simulink library "WECSim_Lib"  (R2014b)
settings: Solver=ode45  StartTime=0.0  StopTime=10.0  RelTol=1e-3
undefined symbols (not defined in the file): body, constraint, pto, simu, waves, X, Y, Z
libraries: nesl_utility x178, sm_lib x59, vrlib x12
(part 3 of 6)

== system WECSim_Lib/PTOs/Translational PTO (Local X) ==
  note: pto.loc
      | pto.c
      | pto.k
  note: Constraints the motion to the desired DOF.
      | Applies PTO loads to the body based on PTO restoring and damping values.
      | Moves the connection points (B and F) from the free surface to the PTO location.
      | Calculates the PTO internal mecahnics force and power.
      | Outputs motions, forces, and power.
  Assignment{,1..3} (4 alike) : Assignment  DiagnosticForDimensions=Warning
  "Assignment (1st index) " : Assignment
  Assignment (1st index)1 : Assignment
  Assignment (1st index)2 : Assignment
  Assignment (1st index)3 : Assignment
  Bus Creator1 : BusCreator  Inputs=8
  Constant{,1..3} (4 alike) : Constant  Value=[0 0 0 0 0 0]
  ForceAndPower : Subsystem
  Gai1 : Gain  Gain=-1
  Gai57 : Gain  Gain=-1
  Gain4 : Gain  Gain=-1
  Gain5 : Gain  Gain=-1
  Mux1 : Mux  Inputs=2
  Mux3 : Mux  Inputs=2
  PS-Simulink Converter{,1..7} (8 alike) : nesl_utility/PS-Simulink Converter  PhysicalDomain=network_engine_domain  SubClassName=ps_output  LeftPortType=input  RightPortType=output  PseudoPeriodic=off  Frequencies=[]  Unit=1  AffineConversion=off
  Rigid Transform : sm_lib/Frames and Transforms/Rigid Transform  TranslationMethod=Cartesian  TranslationLengthUnit=m  TranslationStandardAxis=+Z  TranslationStandardOffset=0  TranslationCartesianOffset=pto.loc  TranslationROffset=0  TranslationROffsetUnits=m  TranslationZOffset=0  TranslationZOffsetUnits=m  TranslationThetaOffset=0  TranslationThetaOffsetUnits=deg  RotationMethod=StandardAxis  RotationAngleUnits=deg  RotationStandardAxis=+Y  RotationAngle=90  RotationArbitraryAxis=[0 0 1]  FollAlignAxisA=+X  BaseAlignAxisA=+Y  FollAlignAxisB=+Y  BaseAlignAxisB=+Z  RotationMatrix=[1 0 0; 0 1 0; 0 0 1]  BlockFunction=simmechanics.library.frames_transforms.rigid_transform
  Rigid Transform1 : sm_lib/Frames and Transforms/Rigid Transform  TranslationMethod=Cartesian  TranslationLengthUnit=m  TranslationStandardAxis=+Z  TranslationStandardOffset=0  TranslationCartesianOffset=pto.loc  TranslationROffset=0  TranslationROffsetUnits=m  TranslationZOffset=0  TranslationZOffsetUnits=m  TranslationThetaOffset=0  TranslationThetaOffsetUnits=deg  RotationMethod=StandardAxis  RotationAngleUnits=deg  RotationStandardAxis=+Y  RotationAngle=90  RotationArbitraryAxis=[0 0 1]  FollAlignAxisA=+X  BaseAlignAxisA=+Y  FollAlignAxisB=+Y  BaseAlignAxisB=+Z  RotationMatrix=[1 0 0; 0 1 0; 0 0 1]  BlockFunction=simmechanics.library.frames_transforms.rigid_transform
  Selector{,2,4,6} (4 alike) : Selector  InputPortWidth=3  Indices=[3 2 1]
  Selector{1,3,5,7} (4 alike) : Selector  InputPortWidth=3  Indices=[3]
  Translational PCC (Prismatic Joint) : sm_lib/Joints/Prismatic Joint  SenseConstraintForce=on  SenseConstraintForceX=off  SenseConstraintForceY=off  SenseConstraintForceZ=off  SenseConstraintTorque=on  SenseConstraintTorqueX=off  SenseConstraintTorqueY=off  SenseConstraintTorqueZ=off  SenseTotalForce=on  SenseTotalForceX=off  SenseTotalForceY=off  SenseTotalForceZ=off  SenseTotalTorque=on  SenseTotalTorqueX=off  SenseTotalTorqueY=off  SenseTotalTorqueZ=off  CompositeWrenchDir=BaseOnFollower  CompositeWrenchFrame=BaseFrame  EquilibriumPosition=0  EquilibriumPositionUnits=m  SpringStiffness=pto.k  SpringStiffnessUnits=N/m  DampingCoefficient=pto.c  DampingCoefficientUnits=N/(m/s)  TorqueActuationMode=NoTorque  MotionActuationMode=ComputedMotion  SensePosition=on  SenseVelocity=on  SenseAcceleration=on  SenseTorqueForce=on  PositionTargetValue=0  PositionTargetValueUnits=m  PositionTargetSpecify=off  PositionTargetPriority=High  VelocityTargetValue=0  VelocityTargetValueUnits=m/s  VelocityTargetSpecify=off  VelocityTargetPriority=High  BlockFunction=simmechanics.library.joints.prismatic_joint
  output : ToWorkspace  VariableName=pto1_out  SaveFormat=Structure With Time  SampleTime=-1
      settings: Decimation=round(simu.dtOut/simu.dt,0)
  F : PMIOPort  Port=1  Side=Left
  B : PMIOPort  Port=2  Side=Right
  wires:
  Selector2/1 -> Selector3/1, Assignment/1
  Selector3/1 -> Gai57/1
  Gai57/1 -> Assignment/2
  Selector/1 -> Selector1/1, Assignment1/1
  Selector1/1 -> Gain4/1
  Gain4/1 -> Assignment1/2
  ForceAndPower/2(Power) -> Bus Creator1/8  "powerInternalMechanics"
  ForceAndPower/1(Force) -> Bus Creator1/7  "forceInternalMechanics"
  Assignment (1st index)2/1 -> Bus Creator1/3  "acceleration"
  Assignment (1st index)1/1 -> ForceAndPower/2(Vel), Bus Creator1/2  "velocity"
  "Assignment (1st index) "/1 -> ForceAndPower/1(Pos), Bus Creator1/1  "position"
  Assignment (1st index)3/1 -> Bus Creator1/5  "forceActuation"
  Mux3/1 -> Bus Creator1/4  "forceTotal"
  Mux1/1 -> Bus Creator1/6  "forceConstraint"
  Bus Creator1/1 -> output/1
  PS-Simulink Converter4/1 -> Selector/1
  PS-Simulink Converter5/1 -> Selector2/1
  Constant/1 -> "Assignment (1st index) "/1
  PS-Simulink Converter/1 -> "Assignment (1st index) "/2
  Constant1/1 -> Assignment (1st index)1/1
  PS-Simulink Converter1/1 -> Assignment (1st index)1/2
  Constant2/1 -> Assignment (1st index)2/1
  Constant3/1 -> Assignment (1st index)3/1
  PS-Simulink Converter2/1 -> Assignment (1st index)2/2
  PS-Simulink Converter3/1 -> Assignment (1st index)3/2
  Assignment1/1 -> Mux1/1
  Assignment/1 -> Mux1/2
  Selector6/1 -> Assignment2/1, Selector7/1
  Selector7/1 -> Gai1/1
  Gai1/1 -> Assignment2/2
  Selector4/1 -> Assignment3/1, Selector5/1
  Selector5/1 -> Gain5/1
  Gain5/1 -> Assignment3/2
  PS-Simulink Converter6/1 -> Selector4/1
  PS-Simulink Converter7/1 -> Selector6/1
  Assignment3/1 -> Mux3/1
  Assignment2/1 -> Mux3/2
  connections:
  Rigid Transform/LConn1 -- B/RConn1
  Rigid Transform/RConn1 -- Translational PCC (Prismatic Joint)/LConn1
  Rigid Transform1/LConn1 -- F/RConn1
  PS-Simulink Converter4/LConn1 -- Translational PCC (Prismatic Joint)/RConn6
  PS-Simulink Converter5/LConn1 -- Translational PCC (Prismatic Joint)/RConn7
  Translational PCC (Prismatic Joint)/RConn2 -- PS-Simulink Converter/LConn1
  Translational PCC (Prismatic Joint)/RConn3 -- PS-Simulink Converter1/LConn1
  Translational PCC (Prismatic Joint)/RConn4 -- PS-Simulink Converter2/LConn1
  Translational PCC (Prismatic Joint)/RConn1 -- Rigid Transform1/RConn1
  Translational PCC (Prismatic Joint)/RConn5 -- PS-Simulink Converter3/LConn1
  Translational PCC (Prismatic Joint)/RConn8 -- PS-Simulink Converter6/LConn1
  PS-Simulink Converter7/LConn1 -- Translational PCC (Prismatic Joint)/RConn9

== system WECSim_Lib/PTOs/Translational PTO (Local Z) ==
  note: pto.loc
      | pto.c
      | pto.k
  note: Constraints the motion to the desired DOF.
      | Applies PTO loads to the body based on PTO restoring and damping values.
      | Moves the connection points (B and F) from the free surface to the PTO location.
      | Calculates the PTO internal mecahnics force and power.
      | Outputs motions, forces, and power.
  "Assignment (3rd index) " : Assignment  Indices=3
  Assignment (3rd index)1 : Assignment  Indices=3
  Assignment (3rd index)2 : Assignment  Indices=3
  Assignment (3rd index)3 : Assignment  Indices=3
  Bus Creator1 : BusCreator  Inputs=8
  Constant{,1..3} (4 alike) : Constant  Value=[0 0 0 0 0 0]
  InternalMechanics : Subsystem
  Mux1 : Mux  Inputs=2
  Mux4 : Mux  Inputs=2
  PS-Simulink Converter{,1..7} (8 alike) : nesl_utility/PS-Simulink Converter  PhysicalDomain=network_engine_domain  SubClassName=ps_output  LeftPortType=input  RightPortType=output  PseudoPeriodic=off  Frequencies=[]  Unit=1  AffineConversion=off
  Rigid Transform : sm_lib/Frames and Transforms/Rigid Transform  TranslationMethod=Cartesian  TranslationLengthUnit=m  TranslationStandardAxis=+Z  TranslationStandardOffset=0  TranslationCartesianOffset=pto.loc  TranslationROffset=0  TranslationROffsetUnits=m  TranslationZOffset=0  TranslationZOffsetUnits=m  TranslationThetaOffset=0  TranslationThetaOffsetUnits=deg  RotationMethod=None  RotationAngleUnits=deg  RotationStandardAxis=+X  RotationAngle=90  RotationArbitraryAxis=[0 0 1]  FollAlignAxisA=+X  BaseAlignAxisA=+Y  FollAlignAxisB=+Y  BaseAlignAxisB=+Z  RotationMatrix=[1 0 0; 0 1 0; 0 0 1]  BlockFunction=simmechanics.library.frames_transforms.rigid_transform
  Rigid Transform1 : sm_lib/Frames and Transforms/Rigid Transform  TranslationMethod=Cartesian  TranslationLengthUnit=m  TranslationStandardAxis=+Z  TranslationStandardOffset=0  TranslationCartesianOffset=pto.loc  TranslationROffset=0  TranslationROffsetUnits=m  TranslationZOffset=0  TranslationZOffsetUnits=m  TranslationThetaOffset=0  TranslationThetaOffsetUnits=deg  RotationMethod=None  RotationAngleUnits=deg  RotationStandardAxis=+X  RotationAngle=90  RotationArbitraryAxis=[0 0 1]  FollAlignAxisA=+X  BaseAlignAxisA=+Y  FollAlignAxisB=+Y  BaseAlignAxisB=+Z  RotationMatrix=[1 0 0; 0 1 0; 0 0 1]  BlockFunction=simmechanics.library.frames_transforms.rigid_transform
  Translational PCC (Prismatic Joint) : sm_lib/Joints/Prismatic Joint  SenseConstraintForce=on  SenseConstraintForceX=off  SenseConstraintForceY=off  SenseConstraintForceZ=off  SenseConstraintTorque=on  SenseConstraintTorqueX=off  SenseConstraintTorqueY=off  SenseConstraintTorqueZ=off  SenseTotalForce=on  SenseTotalForceX=off  SenseTotalForceY=off  SenseTotalForceZ=off  SenseTotalTorque=on  SenseTotalTorqueX=off  SenseTotalTorqueY=off  SenseTotalTorqueZ=off  CompositeWrenchDir=BaseOnFollower  CompositeWrenchFrame=BaseFrame  EquilibriumPosition=0  EquilibriumPositionUnits=m  SpringStiffness=pto.k  SpringStiffnessUnits=N/m  DampingCoefficient=pto.c  DampingCoefficientUnits=N/(m/s)  TorqueActuationMode=NoTorque  MotionActuationMode=ComputedMotion  SensePosition=on  SenseVelocity=on  SenseAcceleration=on  SenseTorqueForce=on  PositionTargetValue=0  PositionTargetValueUnits=m  PositionTargetSpecify=off  PositionTargetPriority=High  VelocityTargetValue=0  VelocityTargetValueUnits=m/s  VelocityTargetSpecify=off  VelocityTargetPriority=High  BlockFunction=simmechanics.library.joints.prismatic_joint
  output : ToWorkspace  VariableName=pto1_out  SaveFormat=Structure With Time  SampleTime=-1
      settings: Decimation=round(simu.dtOut/simu.dt,0)
  F : PMIOPort  Port=1  Side=Left
  B : PMIOPort  Port=2  Side=Right
  wires:
  Bus Creator1/1 -> output/1
  Mux1/1 -> Bus Creator1/6  "forceConstraint"
  Mux4/1 -> Bus Creator1/4  "forceTotal"
  PS-Simulink Converter4/1 -> Mux1/1
  PS-Simulink Converter5/1 -> Mux1/2
  PS-Simulink Converter6/1 -> Mux4/1
  PS-Simulink Converter7/1 -> Mux4/2
  Assignment (3rd index)3/1 -> Bus Creator1/5  "forceActuation"
  "Assignment (3rd index) "/1 -> InternalMechanics/1(Position), Bus Creator1/1  "position"
  Assignment (3rd index)1/1 -> InternalMechanics/2(Velocity), Bus Creator1/2  "velocity"
  Assignment (3rd index)2/1 -> Bus Creator1/3  "acceleration"
  Constant/1 -> "Assignment (3rd index) "/1
  PS-Simulink Converter/1 -> "Assignment (3rd index) "/2
  Constant1/1 -> Assignment (3rd index)1/1
  PS-Simulink Converter1/1 -> Assignment (3rd index)1/2
  Constant2/1 -> Assignment (3rd index)2/1
  PS-Simulink Converter2/1 -> Assignment (3rd index)2/2
  InternalMechanics/1(Force) -> Bus Creator1/7  "forceInternalMechanics"
  InternalMechanics/2(Power) -> Bus Creator1/8  "powerInternalMechanics"
  Constant3/1 -> Assignment (3rd index)3/1
  PS-Simulink Converter3/1 -> Assignment (3rd index)3/2  "forceActuation"
  connections:
  Rigid Transform/RConn1 -- Translational PCC (Prismatic Joint)/LConn1
  B/RConn1 -- Rigid Transform/LConn1
  Translational PCC (Prismatic Joint)/RConn5 -- PS-Simulink Converter3/LConn1
  Translational PCC (Prismatic Joint)/RConn9 -- PS-Simulink Converter7/LConn1
  Translational PCC (Prismatic Joint)/RConn1 -- Rigid Transform1/RConn1
  Translational PCC (Prismatic Joint)/RConn4 -- PS-Simulink Converter2/LConn1
  Translational PCC (Prismatic Joint)/RConn7 -- PS-Simulink Converter5/LConn1
  Translational PCC (Prismatic Joint)/RConn3 -- PS-Simulink Converter1/LConn1
  Rigid Transform1/LConn1 -- F/RConn1
  Translational PCC (Prismatic Joint)/RConn8 -- PS-Simulink Converter6/LConn1
  Translational PCC (Prismatic Joint)/RConn2 -- PS-Simulink Converter/LConn1
  Translational PCC (Prismatic Joint)/RConn6 -- PS-Simulink Converter4/LConn1

== system WECSim_Lib/PTOs/Translational PTO Prescribed Motion (Local X) ==
  note: Constraints the motion to the desired DOF.
      | Applies PTO loads to the body based on PTO restoring and damping values.
      | Additionally forces User Defined motions, and outputs required actuation force.
      | Moves the connection points (B and F) from the free surface to the PTO location.
      | Calculates the PTO internal mecahnics force and power.
      | Outputs motions, forces, and power.
  note: pto.loc
      | pto.c
      | pto.k
  position : Inport
  velocity : Inport  Port=2
  acceleration : Inport  Port=3
  Assignment{,1..3} (4 alike) : Assignment  DiagnosticForDimensions=Warning
  "Assignment (1st index) " : Assignment
  Assignment (1st index)1 : Assignment
  Assignment (1st index)2 : Assignment
  Assignment (1st index)3 : Assignment
  Bus Creator1 : BusCreator  Inputs=8
  Constant{,1..3} (4 alike) : Constant  Value=[0 0 0 0 0 0]
  ForceAndPower : Subsystem
  Gai1 : Gain  Gain=-1
  Gai57 : Gain  Gain=-1
  Gain4 : Gain  Gain=-1
  Gain5 : Gain  Gain=-1
  Mux1 : Mux  Inputs=2
  Mux3 : Mux  Inputs=2
  PS-Simulink Converter{,1..7} (8 alike) : nesl_utility/PS-Simulink Converter  PhysicalDomain=network_engine_domain  SubClassName=ps_output  LeftPortType=input  RightPortType=output  PseudoPeriodic=off  Frequencies=[]  Unit=1  AffineConversion=off
  Rigid Transform : sm_lib/Frames and Transforms/Rigid Transform  TranslationMethod=Cartesian  TranslationLengthUnit=m  TranslationStandardAxis=+Z  TranslationStandardOffset=0  TranslationCartesianOffset=pto.loc  TranslationROffset=0  TranslationROffsetUnits=m  TranslationZOffset=0  TranslationZOffsetUnits=m  TranslationThetaOffset=0  TranslationThetaOffsetUnits=deg  RotationMethod=StandardAxis  RotationAngleUnits=deg  RotationStandardAxis=+Y  RotationAngle=90  RotationArbitraryAxis=[0 0 1]  FollAlignAxisA=+X  BaseAlignAxisA=+Y  FollAlignAxisB=+Y  BaseAlignAxisB=+Z  RotationMatrix=[1 0 0; 0 1 0; 0 0 1]  BlockFunction=simmechanics.library.frames_transforms.rigid_transform
  Rigid Transform1 : sm_lib/Frames and Transforms/Rigid Transform  TranslationMethod=Cartesian  TranslationLengthUnit=m  TranslationStandardAxis=+Z  TranslationStandardOffset=0  TranslationCartesianOffset=pto.loc  TranslationROffset=0  TranslationROffsetUnits=m  TranslationZOffset=0  TranslationZOffsetUnits=m  TranslationThetaOffset=0  TranslationThetaOffsetUnits=deg  RotationMethod=StandardAxis  RotationAngleUnits=deg  RotationStandardAxis=+Y  RotationAngle=90  RotationArbitraryAxis=[0 0 1]  FollAlignAxisA=+X  BaseAlignAxisA=+Y  FollAlignAxisB=+Y  BaseAlignAxisB=+Z  RotationMatrix=[1 0 0; 0 1 0; 0 0 1]  BlockFunction=simmechanics.library.frames_transforms.rigid_transform
  Selector{,2,4,6} (4 alike) : Selector  InputPortWidth=3  Indices=[3 2 1]
  Selector{1,3,5,7} (4 alike) : Selector  InputPortWidth=3  Indices=[3]
  Simulink-PS Converter : nesl_utility/Simulink-PS Converter  PhysicalDomain=network_engine_domain  SubClassName=ps_input  LeftPortType=input  RightPortType=output  PseudoPeriodic=off  Frequencies=[]  NoiseDistribution=none  NoiseParameters=[]  Unit=1  AffineConversion=off  InputFiltering=derivs  SimscapeFilterOrder=2  InputFilterTimeConstant=0.001  UdotUserProvided=2
  Translational PCC (Prismatic Joint) : sm_lib/Joints/Prismatic Joint  SenseConstraintForce=on  SenseConstraintForceX=off  SenseConstraintForceY=off  SenseConstraintForceZ=off  SenseConstraintTorque=on  SenseConstraintTorqueX=off  SenseConstraintTorqueY=off  SenseConstraintTorqueZ=off  SenseTotalForce=on  SenseTotalForceX=off  SenseTotalForceY=off  SenseTotalForceZ=off  SenseTotalTorque=on  SenseTotalTorqueX=off  SenseTotalTorqueY=off  SenseTotalTorqueZ=off  CompositeWrenchDir=BaseOnFollower  CompositeWrenchFrame=BaseFrame  EquilibriumPosition=0  EquilibriumPositionUnits=m  SpringStiffness=pto.k  SpringStiffnessUnits=N/m  DampingCoefficient=pto.c  DampingCoefficientUnits=N/(m/s)  TorqueActuationMode=ComputedTorque  MotionActuationMode=InputMotion  SensePosition=on  SenseVelocity=on  SenseAcceleration=on  SenseTorqueForce=on  PositionTargetValue=0  PositionTargetValueUnits=m  PositionTargetSpecify=off  PositionTargetPriority=High  VelocityTargetValue=0  VelocityTargetValueUnits=m/s  VelocityTargetSpecify=off  VelocityTargetPriority=High  BlockFunction=simmechanics.library.joints.prismatic_joint
  output : ToWorkspace  VariableName=pto1_out  SaveFormat=Structure With Time  SampleTime=-1
      settings: Decimation=round(simu.dtOut/simu.dt,0)
  F : PMIOPort  Port=1  Side=Left
  B : PMIOPort  Port=2  Side=Right
  wires:
  acceleration/1 -> Simulink-PS Converter/3
  velocity/1 -> Simulink-PS Converter/2
  position/1 -> Simulink-PS Converter/1
  Assignment2/1 -> Mux3/2
  Assignment3/1 -> Mux3/1
  PS-Simulink Converter7/1 -> Selector6/1
  PS-Simulink Converter6/1 -> Selector4/1
  Gain5/1 -> Assignment3/2
  Selector5/1 -> Gain5/1
  Selector4/1 -> Selector5/1, Assignment3/1
  Gai1/1 -> Assignment2/2
  Selector7/1 -> Gai1/1
  Selector6/1 -> Selector7/1, Assignment2/1
  Assignment/1 -> Mux1/2
  Assignment1/1 -> Mux1/1
  PS-Simulink Converter3/1 -> Assignment (1st index)3/2
  PS-Simulink Converter2/1 -> Assignment (1st index)2/2
  Constant3/1 -> Assignment (1st index)3/1
  Constant2/1 -> Assignment (1st index)2/1
  PS-Simulink Converter1/1 -> Assignment (1st index)1/2
  Constant1/1 -> Assignment (1st index)1/1
  PS-Simulink Converter/1 -> "Assignment (1st index) "/2
  Constant/1 -> "Assignment (1st index) "/1
  PS-Simulink Converter5/1 -> Selector2/1
  PS-Simulink Converter4/1 -> Selector/1
  Bus Creator1/1 -> output/1
  Mux1/1 -> Bus Creator1/6  "forceConstraint"
  Mux3/1 -> Bus Creator1/4  "forceTotal"
  Assignment (1st index)3/1 -> Bus Creator1/5  "forceActuation"
  ForceAndPower/1(Force) -> Bus Creator1/7  "forceInternalMechanics"
  ForceAndPower/2(Power) -> Bus Creator1/8  "powerInternalMechanics"
  Gain4/1 -> Assignment1/2
  Selector1/1 -> Gain4/1
  Selector/1 -> Assignment1/1, Selector1/1
  Gai57/1 -> Assignment/2
  Selector3/1 -> Gai57/1
  Selector2/1 -> Assignment/1, Selector3/1
  "Assignment (1st index) "/1 -> ForceAndPower/1(Pos), Bus Creator1/1  "position"
  Assignment (1st index)1/1 -> ForceAndPower/2(Vel), Bus Creator1/2  "velocity"
  Assignment (1st index)2/1 -> Bus Creator1/3  "acceleration"
  connections:
  Simulink-PS Converter/RConn1 -- Translational PCC (Prismatic Joint)/LConn2
  PS-Simulink Converter7/LConn1 -- Translational PCC (Prismatic Joint)/RConn9
  Translational PCC (Prismatic Joint)/RConn8 -- PS-Simulink Converter6/LConn1
  Translational PCC (Prismatic Joint)/RConn5 -- PS-Simulink Converter3/LConn1
  Translational PCC (Prismatic Joint)/RConn1 -- Rigid Transform1/RConn1
  Translational PCC (Prismatic Joint)/RConn4 -- PS-Simulink Converter2/LConn1
  Translational PCC (Prismatic Joint)/RConn3 -- PS-Simulink Converter1/LConn1
  Translational PCC (Prismatic Joint)/RConn2 -- PS-Simulink Converter/LConn1
  PS-Simulink Converter5/LConn1 -- Translational PCC (Prismatic Joint)/RConn7
  PS-Simulink Converter4/LConn1 -- Translational PCC (Prismatic Joint)/RConn6
  Rigid Transform1/LConn1 -- F/RConn1
  Rigid Transform/RConn1 -- Translational PCC (Prismatic Joint)/LConn1
  Rigid Transform/LConn1 -- B/RConn1

== system WECSim_Lib/PTOs/Translational PTO Prescribed Motion (Local Z) ==
  note: Constraints the motion to the desired DOF.
      | Applies PTO loads to the body based on PTO restoring and damping values.
      | Additionally forces User Defined motions, and outputs required actuation force.
      | Moves the connection points (B and F) from the free surface to the PTO location.
      | Calculates the PTO internal mecahnics force and power.
      | Outputs motions, forces, and power.
  note: pto.loc
      | pto.c
      | pto.k
  position : Inport
  velocity : Inport  Port=2
  acceleration : Inport  Port=3
  "Assignment (3rd index) " : Assignment  Indices=3
  Assignment (3rd index)1 : Assignment  Indices=3
  Assignment (3rd index)2 : Assignment  Indices=3
  Assignment (3rd index)3 : Assignment  Indices=3
  Bus Creator1 : BusCreator  Inputs=8
  Constant{,1..3} (4 alike) : Constant  Value=[0 0 0 0 0 0]
  InternalMechanics : Subsystem
  Mux1 : Mux  Inputs=2
  Mux4 : Mux  Inputs=2
  PS-Simulink Converter{,1..7} (8 alike) : nesl_utility/PS-Simulink Converter  PhysicalDomain=network_engine_domain  SubClassName=ps_output  LeftPortType=input  RightPortType=output  PseudoPeriodic=off  Frequencies=[]  Unit=1  AffineConversion=off
  Rigid Transform : sm_lib/Frames and Transforms/Rigid Transform  TranslationMethod=Cartesian  TranslationLengthUnit=m  TranslationStandardAxis=+Z  TranslationStandardOffset=0  TranslationCartesianOffset=pto.loc  TranslationROffset=0  TranslationROffsetUnits=m  TranslationZOffset=0  TranslationZOffsetUnits=m  TranslationThetaOffset=0  TranslationThetaOffsetUnits=deg  RotationMethod=None  RotationAngleUnits=deg  RotationStandardAxis=+X  RotationAngle=90  RotationArbitraryAxis=[0 0 1]  FollAlignAxisA=+X  BaseAlignAxisA=+Y  FollAlignAxisB=+Y  BaseAlignAxisB=+Z  RotationMatrix=[1 0 0; 0 1 0; 0 0 1]  BlockFunction=simmechanics.library.frames_transforms.rigid_transform
  Rigid Transform1 : sm_lib/Frames and Transforms/Rigid Transform  TranslationMethod=Cartesian  TranslationLengthUnit=m  TranslationStandardAxis=+Z  TranslationStandardOffset=0  TranslationCartesianOffset=pto.loc  TranslationROffset=0  TranslationROffsetUnits=m  TranslationZOffset=0  TranslationZOffsetUnits=m  TranslationThetaOffset=0  TranslationThetaOffsetUnits=deg  RotationMethod=None  RotationAngleUnits=deg  RotationStandardAxis=+X  RotationAngle=90  RotationArbitraryAxis=[0 0 1]  FollAlignAxisA=+X  BaseAlignAxisA=+Y  FollAlignAxisB=+Y  BaseAlignAxisB=+Z  RotationMatrix=[1 0 0; 0 1 0; 0 0 1]  BlockFunction=simmechanics.library.frames_transforms.rigid_transform
  Simulink-PS Converter : nesl_utility/Simulink-PS Converter  PhysicalDomain=network_engine_domain  SubClassName=ps_input  LeftPortType=input  RightPortType=output  PseudoPeriodic=off  Frequencies=[]  NoiseDistribution=none  NoiseParameters=[]  Unit=1  AffineConversion=off  InputFiltering=derivs  SimscapeFilterOrder=2  InputFilterTimeConstant=0.001  UdotUserProvided=2
  Translational PCC (Prismatic Joint) : sm_lib/Joints/Prismatic Joint  SenseConstraintForce=on  SenseConstraintForceX=off  SenseConstraintForceY=off  SenseConstraintForceZ=off  SenseConstraintTorque=on  SenseConstraintTorqueX=off  SenseConstraintTorqueY=off  SenseConstraintTorqueZ=off  SenseTotalForce=on  SenseTotalForceX=off  SenseTotalForceY=off  SenseTotalForceZ=off  SenseTotalTorque=on  SenseTotalTorqueX=off  SenseTotalTorqueY=off  SenseTotalTorqueZ=off  CompositeWrenchDir=BaseOnFollower  CompositeWrenchFrame=BaseFrame  EquilibriumPosition=0  EquilibriumPositionUnits=m  SpringStiffness=pto.k  SpringStiffnessUnits=N/m  DampingCoefficient=pto.c  DampingCoefficientUnits=N/(m/s)  TorqueActuationMode=ComputedTorque  MotionActuationMode=InputMotion  SensePosition=on  SenseVelocity=on  SenseAcceleration=on  SenseTorqueForce=on  PositionTargetValue=0  PositionTargetValueUnits=m  PositionTargetSpecify=off  PositionTargetPriority=High  VelocityTargetValue=0  VelocityTargetValueUnits=m/s  VelocityTargetSpecify=off  VelocityTargetPriority=High  BlockFunction=simmechanics.library.joints.prismatic_joint
  output : ToWorkspace  VariableName=pto1_out  SaveFormat=Structure With Time  SampleTime=-1
      settings: Decimation=round(simu.dtOut/simu.dt,0)
  F : PMIOPort  Port=1  Side=Left
  B : PMIOPort  Port=2  Side=Right
  wires:
  acceleration/1 -> Simulink-PS Converter/3
  velocity/1 -> Simulink-PS Converter/2
  position/1 -> Simulink-PS Converter/1
  Bus Creator1/1 -> output/1
  Mux1/1 -> Bus Creator1/6  "forceConstraint"
  Mux4/1 -> Bus Creator1/4  "forceTotal"
  PS-Simulink Converter4/1 -> Mux1/1
  PS-Simulink Converter5/1 -> Mux1/2
  PS-Simulink Converter6/1 -> Mux4/1
  PS-Simulink Converter7/1 -> Mux4/2
  Assignment (3rd index)3/1 -> Bus Creator1/5  "forceActuation"
  "Assignment (3rd index) "/1 -> InternalMechanics/1(Position), Bus Creator1/1  "position"
  Assignment (3rd index)1/1 -> InternalMechanics/2(Velocity), Bus Creator1/2  "velocity"
  Assignment (3rd index)2/1 -> Bus Creator1/3  "acceleration"
  Constant/1 -> "Assignment (3rd index) "/1
  PS-Simulink Converter/1 -> "Assignment (3rd index) "/2
  Constant1/1 -> Assignment (3rd index)1/1
  PS-Simulink Converter1/1 -> Assignment (3rd index)1/2
  Constant2/1 -> Assignment (3rd index)2/1
  PS-Simulink Converter2/1 -> Assignment (3rd index)2/2
  InternalMechanics/1(Force) -> Bus Creator1/7  "forceInternalMechanics"
  InternalMechanics/2(Power) -> Bus Creator1/8  "powerInternalMechanics"
  Constant3/1 -> Assignment (3rd index)3/1
  PS-Simulink Converter3/1 -> Assignment (3rd index)3/2  "forceActuation"
  connections:
  Translational PCC (Prismatic Joint)/LConn2 -- Simulink-PS Converter/RConn1
  Rigid Transform1/LConn1 -- F/RConn1
  Translational PCC (Prismatic Joint)/RConn1 -- Rigid Transform1/RConn1
  Rigid Transform/RConn1 -- Translational PCC (Prismatic Joint)/LConn1
  B/RConn1 -- Rigid Transform/LConn1
  Translational PCC (Prismatic Joint)/RConn2 -- PS-Simulink Converter/LConn1
  Translational PCC (Prismatic Joint)/RConn3 -- PS-Simulink Converter1/LConn1
  Translational PCC (Prismatic Joint)/RConn4 -- PS-Simulink Converter2/LConn1
  Translational PCC (Prismatic Joint)/RConn5 -- PS-Simulink Converter3/LConn1
  Translational PCC (Prismatic Joint)/RConn6 -- PS-Simulink Converter4/LConn1
  Translational PCC (Prismatic Joint)/RConn7 -- PS-Simulink Converter5/LConn1
  Translational PCC (Prismatic Joint)/RConn8 -- PS-Simulink Converter6/LConn1
  Translational PCC (Prismatic Joint)/RConn9 -- PS-Simulink Converter7/LConn1

== system WECSim_Lib/PTOs/Translational PTO UD Force (Local X) ==
  note: Constraints the motion to the desired DOF.
      | Applies PTO loads to the body based on PTO restoring and damping values.
      | Additionally applies user defined PTO force and outputs PTO position,velocity and acceleration.
      | Moves the connection points (B and F) from the free surface to the PTO location.
      | Calculates the PTO internal mecahnics force and power.
      | Outputs motions, forces, and power.
  note: pto.loc
      | pto.c
      | pto.k
  Torque : Inport
  Assignment{,1..3} (4 alike) : Assignment  DiagnosticForDimensions=Warning
  "Assignment (1st index) " : Assignment
  Assignment (1st index)1 : Assignment
  Assignment (1st index)2 : Assignment
  Assignment (1st index)3 : Assignment
  Bus Creator1 : BusCreator  Inputs=8
  Bus Creator2 : BusCreator  Inputs=3
  Constant{,1..3} (4 alike) : Constant  Value=[0 0 0 0 0 0]
  ForceAndPower : Subsystem
  Gai1 : Gain  Gain=-1
  Gai57 : Gain  Gain=-1
  Gain4 : Gain  Gain=-1
  Gain5 : Gain  Gain=-1
  Mux1 : Mux  Inputs=2
  Mux3 : Mux  Inputs=2
  PS-Simulink Converter{,1..7} (8 alike) : nesl_utility/PS-Simulink Converter  PhysicalDomain=network_engine_domain  SubClassName=ps_output  LeftPortType=input  RightPortType=output  PseudoPeriodic=off  Frequencies=[]  Unit=1  AffineConversion=off
  Rigid Transform : sm_lib/Frames and Transforms/Rigid Transform  TranslationMethod=Cartesian  TranslationLengthUnit=m  TranslationStandardAxis=+Z  TranslationStandardOffset=0  TranslationCartesianOffset=pto.loc  TranslationROffset=0  TranslationROffsetUnits=m  TranslationZOffset=0  TranslationZOffsetUnits=m  TranslationThetaOffset=0  TranslationThetaOffsetUnits=deg  RotationMethod=StandardAxis  RotationAngleUnits=deg  RotationStandardAxis=+Y  RotationAngle=90  RotationArbitraryAxis=[0 0 1]  FollAlignAxisA=+X  BaseAlignAxisA=+Y  FollAlignAxisB=+Y  BaseAlignAxisB=+Z  RotationMatrix=[1 0 0; 0 1 0; 0 0 1]  BlockFunction=simmechanics.library.frames_transforms.rigid_transform
  Rigid Transform1 : sm_lib/Frames and Transforms/Rigid Transform  TranslationMethod=Cartesian  TranslationLengthUnit=m  TranslationStandardAxis=+Z  TranslationStandardOffset=0  TranslationCartesianOffset=pto.loc  TranslationROffset=0  TranslationROffsetUnits=m  TranslationZOffset=0  TranslationZOffsetUnits=m  TranslationThetaOffset=0  TranslationThetaOffsetUnits=deg  RotationMethod=StandardAxis  RotationAngleUnits=deg  RotationStandardAxis=+Y  RotationAngle=90  RotationArbitraryAxis=[0 0 1]  FollAlignAxisA=+X  BaseAlignAxisA=+Y  FollAlignAxisB=+Y  BaseAlignAxisB=+Z  RotationMatrix=[1 0 0; 0 1 0; 0 0 1]  BlockFunction=simmechanics.library.frames_transforms.rigid_transform
  Selector{,2,4,6} (4 alike) : Selector  InputPortWidth=3  Indices=[3 2 1]
  Selector{1,3,5,7} (4 alike) : Selector  InputPortWidth=3  Indices=[3]
  Simulink-PS Converter : nesl_utility/Simulink-PS Converter  PhysicalDomain=network_engine_domain  SubClassName=ps_input  LeftPortType=input  RightPortType=output  PseudoPeriodic=off  Frequencies=[]  NoiseDistribution=none  NoiseParameters=[]  Unit=1  AffineConversion=off  InputFiltering=off  SimscapeFilterOrder=1  InputFilterTimeConstant=0.001  UdotUserProvided=1
  Translational PCC (Prismatic Joint) : sm_lib/Joints/Prismatic Joint  SenseConstraintForce=on  SenseConstraintForceX=off  SenseConstraintForceY=off  SenseConstraintForceZ=off  SenseConstraintTorque=on  SenseConstraintTorqueX=off  SenseConstraintTorqueY=off  SenseConstraintTorqueZ=off  SenseTotalForce=on  SenseTotalForceX=off  SenseTotalForceY=off  SenseTotalForceZ=off  SenseTotalTorque=on  SenseTotalTorqueX=off  SenseTotalTorqueY=off  SenseTotalTorqueZ=off  CompositeWrenchDir=BaseOnFollower  CompositeWrenchFrame=BaseFrame  EquilibriumPosition=0  EquilibriumPositionUnits=m  SpringStiffness=pto.k  SpringStiffnessUnits=N/m  DampingCoefficient=pto.c  DampingCoefficientUnits=N/(m/s)  TorqueActuationMode=InputTorque  MotionActuationMode=ComputedMotion  SensePosition=on  SenseVelocity=on  SenseAcceleration=on  SenseTorqueForce=on  PositionTargetValue=0  PositionTargetValueUnits=m  PositionTargetSpecify=off  PositionTargetPriority=High  VelocityTargetValue=0  VelocityTargetValueUnits=m/s  VelocityTargetSpecify=off  VelocityTargetPriority=High  BlockFunction=simmechanics.library.joints.prismatic_joint
  output : ToWorkspace  VariableName=pto1_out  SaveFormat=Structure With Time  SampleTime=-1
      settings: Decimation=round(simu.dtOut/simu.dt,0)
  F : PMIOPort  Port=1  Side=Left
  B : PMIOPort  Port=2  Side=Right
  Response : Outport
  wires:
  Torque/1 -> Simulink-PS Converter/1
  Assignment (1st index)2/1 -> Bus Creator1/3, Bus Creator2/3  "acceleration"
  Assignment (1st index)1/1 -> Bus Creator1/2, Bus Creator2/2, ForceAndPower/2(Vel)  "velocity"
  "Assignment (1st index) "/1 -> Bus Creator1/1, Bus Creator2/1, ForceAndPower/1(Pos)  "position"
  Bus Creator2/1 -> Response/1
  Selector2/1 -> Selector3/1, Assignment/1
  Selector3/1 -> Gai57/1
  Gai57/1 -> Assignment/2
  Selector/1 -> Selector1/1, Assignment1/1
  Selector1/1 -> Gain4/1
  Gain4/1 -> Assignment1/2
  ForceAndPower/2(Power) -> Bus Creator1/8  "powerInternalMechanics"
  ForceAndPower/1(Force) -> Bus Creator1/7  "forceInternalMechanics"
  Assignment (1st index)3/1 -> Bus Creator1/5  "forceActuation"
  Mux3/1 -> Bus Creator1/4  "forceTotal"
  Mux1/1 -> Bus Creator1/6  "forceConstraint"
  Bus Creator1/1 -> output/1
  PS-Simulink Converter4/1 -> Selector/1
  PS-Simulink Converter5/1 -> Selector2/1
  Constant/1 -> "Assignment (1st index) "/1
  PS-Simulink Converter/1 -> "Assignment (1st index) "/2
  Constant1/1 -> Assignment (1st index)1/1
  PS-Simulink Converter1/1 -> Assignment (1st index)1/2
  Constant2/1 -> Assignment (1st index)2/1
  Constant3/1 -> Assignment (1st index)3/1
  PS-Simulink Converter2/1 -> Assignment (1st index)2/2
  PS-Simulink Converter3/1 -> Assignment (1st index)3/2
  Assignment1/1 -> Mux1/1
  Assignment/1 -> Mux1/2
  Selector6/1 -> Assignment2/1, Selector7/1
  Selector7/1 -> Gai1/1
  Gai1/1 -> Assignment2/2
  Selector4/1 -> Assignment3/1, Selector5/1
  Selector5/1 -> Gain5/1
  Gain5/1 -> Assignment3/2
  PS-Simulink Converter6/1 -> Selector4/1
  PS-Simulink Converter7/1 -> Selector6/1
  Assignment3/1 -> Mux3/1
  Assignment2/1 -> Mux3/2
  connections:
  Simulink-PS Converter/RConn1 -- Translational PCC (Prismatic Joint)/LConn2
  Rigid Transform/LConn1 -- B/RConn1
  Rigid Transform/RConn1 -- Translational PCC (Prismatic Joint)/LConn1
  Rigid Transform1/LConn1 -- F/RConn1
  PS-Simulink Converter4/LConn1 -- Translational PCC (Prismatic Joint)/RConn6
  PS-Simulink Converter5/LConn1 -- Translational PCC (Prismatic Joint)/RConn7
  Translational PCC (Prismatic Joint)/RConn2 -- PS-Simulink Converter/LConn1
  Translational PCC (Prismatic Joint)/RConn3 -- PS-Simulink Converter1/LConn1
  Translational PCC (Prismatic Joint)/RConn4 -- PS-Simulink Converter2/LConn1
  Translational PCC (Prismatic Joint)/RConn1 -- Rigid Transform1/RConn1
  Translational PCC (Prismatic Joint)/RConn5 -- PS-Simulink Converter3/LConn1
  Translational PCC (Prismatic Joint)/RConn8 -- PS-Simulink Converter6/LConn1
  PS-Simulink Converter7/LConn1 -- Translational PCC (Prismatic Joint)/RConn9

== system WECSim_Lib/PTOs/Translational PTO UD Force (Local Z) ==
  note: Constraints the motion to the desired DOF.
      | Applies PTO loads to the body based on PTO restoring and damping values.
      | Additionally applies user defined PTO force and outputs PTO position,velocity and acceleration.
      | Moves the connection points (B and F) from the free surface to the PTO location.
      | Calculates the PTO internal mecahnics force and power.
      | Outputs motions, forces, and power.
  note: pto.loc
      | pto.c
      | pto.k
  Force : Inport
  "Assignment (3rd index) " : Assignment  Indices=3
  Assignment (3rd index)1 : Assignment  Indices=3
  Assignment (3rd index)2 : Assignment  Indices=3
  Assignment (3rd index)3 : Assignment  Indices=3
  Bus Creator1 : BusCreator  Inputs=8
  Bus Creator2 : BusCreator  Inputs=3
  Constant{,1..3} (4 alike) : Constant  Value=[0 0 0 0 0 0]
  InternalMechanics : Subsystem
  Mux1 : Mux  Inputs=2
  Mux4 : Mux  Inputs=2
  PS-Simulink Converter{,1..7} (8 alike) : nesl_utility/PS-Simulink Converter  PhysicalDomain=network_engine_domain  SubClassName=ps_output  LeftPortType=input  RightPortType=output  PseudoPeriodic=off  Frequencies=[]  Unit=1  AffineConversion=off
  Rigid Transform : sm_lib/Frames and Transforms/Rigid Transform  TranslationMethod=Cartesian  TranslationLengthUnit=m  TranslationStandardAxis=+Z  TranslationStandardOffset=0  TranslationCartesianOffset=pto.loc  TranslationROffset=0  TranslationROffsetUnits=m  TranslationZOffset=0  TranslationZOffsetUnits=m  TranslationThetaOffset=0  TranslationThetaOffsetUnits=deg  RotationMethod=None  RotationAngleUnits=deg  RotationStandardAxis=+X  RotationAngle=90  RotationArbitraryAxis=[0 0 1]  FollAlignAxisA=+X  BaseAlignAxisA=+Y  FollAlignAxisB=+Y  BaseAlignAxisB=+Z  RotationMatrix=[1 0 0; 0 1 0; 0 0 1]  BlockFunction=simmechanics.library.frames_transforms.rigid_transform
  Rigid Transform1 : sm_lib/Frames and Transforms/Rigid Transform  TranslationMethod=Cartesian  TranslationLengthUnit=m  TranslationStandardAxis=+Z  TranslationStandardOffset=0  TranslationCartesianOffset=pto.loc  TranslationROffset=0  TranslationROffsetUnits=m  TranslationZOffset=0  TranslationZOffsetUnits=m  TranslationThetaOffset=0  TranslationThetaOffsetUnits=deg  RotationMethod=None  RotationAngleUnits=deg  RotationStandardAxis=+X  RotationAngle=90  RotationArbitraryAxis=[0 0 1]  FollAlignAxisA=+X  BaseAlignAxisA=+Y  FollAlignAxisB=+Y  BaseAlignAxisB=+Z  RotationMatrix=[1 0 0; 0 1 0; 0 0 1]  BlockFunction=simmechanics.library.frames_transforms.rigid_transform
  Simulink-PS Converter : nesl_utility/Simulink-PS Converter  PhysicalDomain=network_engine_domain  SubClassName=ps_input  LeftPortType=input  RightPortType=output  PseudoPeriodic=off  Frequencies=[]  NoiseDistribution=none  NoiseParameters=[]  Unit=1  AffineConversion=off  InputFiltering=off  SimscapeFilterOrder=1  InputFilterTimeConstant=0.001  UdotUserProvided=1
  Translational PCC (Prismatic Joint) : sm_lib/Joints/Prismatic Joint  SenseConstraintForce=on  SenseConstraintForceX=off  SenseConstraintForceY=off  SenseConstraintForceZ=off  SenseConstraintTorque=on  SenseConstraintTorqueX=off  SenseConstraintTorqueY=off  SenseConstraintTorqueZ=off  SenseTotalForce=on  SenseTotalForceX=off  SenseTotalForceY=off  SenseTotalForceZ=off  SenseTotalTorque=on  SenseTotalTorqueX=off  SenseTotalTorqueY=off  SenseTotalTorqueZ=off  CompositeWrenchDir=BaseOnFollower  CompositeWrenchFrame=BaseFrame  EquilibriumPosition=0  EquilibriumPositionUnits=m  SpringStiffness=pto.k  SpringStiffnessUnits=N/m  DampingCoefficient=pto.c  DampingCoefficientUnits=N/(m/s)  TorqueActuationMode=InputTorque  MotionActuationMode=ComputedMotion  SensePosition=on  SenseVelocity=on  SenseAcceleration=on  SenseTorqueForce=on  PositionTargetValue=0  PositionTargetValueUnits=m  PositionTargetSpecify=off  PositionTargetPriority=High  VelocityTargetValue=0  VelocityTargetValueUnits=m/s  VelocityTargetSpecify=off  VelocityTargetPriority=High  BlockFunction=simmechanics.library.joints.prismatic_joint
  output : ToWorkspace  VariableName=pto1_out  SaveFormat=Structure With Time  SampleTime=-1
      settings: Decimation=round(simu.dtOut/simu.dt,0)
  F : PMIOPort  Port=1  Side=Left
  B : PMIOPort  Port=2  Side=Right
  Response : Outport
  wires:
  PS-Simulink Converter3/1 -> Assignment (3rd index)3/2  "forceActuation"
  Constant3/1 -> Assignment (3rd index)3/1
  InternalMechanics/2(Power) -> Bus Creator1/8  "powerInternalMechanics"
  InternalMechanics/1(Force) -> Bus Creator1/7  "forceInternalMechanics"
  PS-Simulink Converter2/1 -> Assignment (3rd index)2/2
  Constant2/1 -> Assignment (3rd index)2/1
  PS-Simulink Converter1/1 -> Assignment (3rd index)1/2
  Constant1/1 -> Assignment (3rd index)1/1
  PS-Simulink Converter/1 -> "Assignment (3rd index) "/2
  Constant/1 -> "Assignment (3rd index) "/1
  Assignment (3rd index)2/1 -> Bus Creator1/3, Bus Creator2/3  "acceleration"
  Assignment (3rd index)1/1 -> InternalMechanics/2(Velocity), Bus Creator1/2, Bus Creator2/2  "velocity"
  "Assignment (3rd index) "/1 -> InternalMechanics/1(Position), Bus Creator1/1, Bus Creator2/1  "position"
  Assignment (3rd index)3/1 -> Bus Creator1/5  "forceActuation"
  PS-Simulink Converter7/1 -> Mux4/2
  PS-Simulink Converter6/1 -> Mux4/1
  PS-Simulink Converter5/1 -> Mux1/2
  PS-Simulink Converter4/1 -> Mux1/1
  Mux4/1 -> Bus Creator1/4  "forceTotal"
  Mux1/1 -> Bus Creator1/6  "forceConstraint"
  Bus Creator2/1 -> Response/1
  Force/1 -> Simulink-PS Converter/1
  Bus Creator1/1 -> output/1
  connections:
  Translational PCC (Prismatic Joint)/RConn9 -- PS-Simulink Converter7/LConn1
  Translational PCC (Prismatic Joint)/RConn8 -- PS-Simulink Converter6/LConn1
  Translational PCC (Prismatic Joint)/RConn7 -- PS-Simulink Converter5/LConn1
  Translational PCC (Prismatic Joint)/RConn6 -- PS-Simulink Converter4/LConn1
  Translational PCC (Prismatic Joint)/RConn5 -- PS-Simulink Converter3/LConn1
  Translational PCC (Prismatic Joint)/RConn4 -- PS-Simulink Converter2/LConn1
  Translational PCC (Prismatic Joint)/RConn3 -- PS-Simulink Converter1/LConn1
  Translational PCC (Prismatic Joint)/RConn2 -- PS-Simulink Converter/LConn1
  Simulink-PS Converter/RConn1 -- Translational PCC (Prismatic Joint)/LConn2
  B/RConn1 -- Rigid Transform/LConn1
  Rigid Transform/RConn1 -- Translational PCC (Prismatic Joint)/LConn1
  Translational PCC (Prismatic Joint)/RConn1 -- Rigid Transform1/RConn1
  Rigid Transform1/LConn1 -- F/RConn1

== system WECSim_Lib/Body Elements/Rigid Body/Additional Linear Damping Force Calculation ==
  note: Calculates the additional linear damping force (if any)
      |
      | Additional Linear Damping Force = damping matrix (diagonal) * velocity vector = C * v
  Velocity : Inport
  Additional Linear Damping Matrix (diagonal) : Constant  Value=body.hydroForce.linearDamping
  Product1 : Product  Multiplication=Matrix(*)
  F_LinearDamping : Outport
  wires:
  Additional Linear Damping Matrix (diagonal)/1 -> Product1/1  "C"
  Product1/1 -> F_LinearDamping/1  "F_LinearDamping"
  Velocity/1 -> Product1/2  "v"

== system WECSim_Lib/Body Elements/Rigid Body/B2B Subsystem ==
  note: 1) Add Subsystem or Model blocks as valid variant choices.
      | 2) You cannot connect blocks at this level. At simulation, connectivity is automatically
      | determined, based on the active variant and port name matching.
  vel_in : Inport
  acc_in : Inport  Port=2
  B2B : Subsystem  VariantControl=sv_B2B
  noB2B : Subsystem  VariantControl=sv_noB2B
  vel : Outport
  acc : Outport  Port=2

== system WECSim_Lib/Body Elements/Rigid Body/Hydrostatic Restoring Force Calculation ==
  Displacement : Inport
  Wave Elv : Inport  Port=2
  Time : Inport  Port=3
  Add : Sum  Inputs=+-
  Center of Gravity : Constant  Value=body.hydroData.properties.cg
  Constant : Constant  Value=[0 0 0]
  Linear and Nonlinear Restoring Force Variant Subsystem : Subsystem  Variant=on
  Mux : Mux  Inputs=2
  F_Restoring : Outport
  wires:
  Displacement/1 -> Add/1  "x"
  Linear and Nonlinear Restoring Force Variant Subsystem/1(Out1) -> F_Restoring/1  "F_Restoring"
  Add/1 -> Linear and Nonlinear Restoring Force Variant Subsystem/1(In1)  "x_cg"
  Mux/1 -> Add/2
  Center of Gravity/1 -> Mux/1  "cg"
  Constant/1 -> Mux/2
  Wave Elv/1 -> Linear and Nonlinear Restoring Force Variant Subsystem/2(In2)
  Time/1 -> Linear and Nonlinear Restoring Force Variant Subsystem/3(In3)

== system WECSim_Lib/Body Elements/Rigid Body/Mooring Force Calculation (Map) ==
  note: Calculates the Mooring Force
      |
      | Mooring force = Kmooring matrix * displacement vector (relative to cg)
      | 	+ Cmooring matrix * velocity vector
      | 	- PreTension vector
      | F_Mooring = x_cg * Km  +  v * Cm  -  T
  Displacement : Inport
  Velocity : Inport  Port=2
  0 Disp for Rotation : Constant  Value=[0 0 0]
  Add : Sum  Inputs=+-
  Center of Gravity : Constant  Value=body.hydroData.properties.cg
  Center of Gravity2 : Constant  Value=body.mooring.c
  Mooring K Matrix : Constant  Value=body.mooring.k
  Mooring Pre-Tension : Constant  Value=body.mooring.preTension
  Mux : Mux  Inputs=2
  Product : Product  Multiplication=Matrix(*)
  Product1 : Product  Multiplication=Matrix(*)
  sum : Sum  Inputs=++-
  F_Mooring : Outport
  wires:
  0 Disp for Rotation/1 -> Mux/2
  Center of Gravity2/1 -> Product1/1  "Cm"
  Velocity/1 -> Product1/2  "v"
  Mooring K Matrix/1 -> Product/1  "Km"
  Center of Gravity/1 -> Mux/1  "cg"
  Displacement/1 -> Add/1  "x"
  Mux/1 -> Add/2
  Add/1 -> Product/2  "x_cg"
  Mooring Pre-Tension/1 -> sum/3  "T"
  sum/1 -> F_Mooring/1  "F_Mooring"
  Product1/1 -> sum/2  "Cm*v"
  Product/1 -> sum/1  "Km*x_cg"

== system WECSim_Lib/Body Elements/Rigid Body/Morrison Element and ViscousDampingForceCalculation ==
  Displacement : Inport
  Acceleration : Inport  Port=2
  Velocity : Inport  Port=3
  Abs1 : Abs
  Morrison Element Variant Subsystem : Subsystem  Variant=on
  Product : Product
  Product1 : Product  Multiplication=Matrix(*)
  Transport Delay : TransportDelay  DelayTime=10e-8
  "VisSum " : Sum
  "Viscous Damping Matrix (diagonal) " : Constant  Value=body.hydroForce.visDrag
  F_MorrisonAndViscous : Outport
  wires:
  Velocity/1 -> Morrison Element Variant Subsystem/2(In2), Product/1, Abs1/1
  "VisSum "/1 -> F_MorrisonAndViscous/1  "F_MorrisonAndViscous"
  Transport Delay/1 -> Morrison Element Variant Subsystem/3(In3)
  Acceleration/1 -> Transport Delay/1
  Abs1/1 -> Product/2
  Product1/1 -> "VisSum "/1
  "Viscous Damping Matrix (diagonal) "/1 -> Product1/1  "0.5 * cd * rho *A"
  Product/1 -> Product1/2  "v * |v|"
  Displacement/1 -> Morrison Element Variant Subsystem/1(In1)
  Morrison Element Variant Subsystem/1(Out1) -> "VisSum "/2

== system WECSim_Lib/Body Elements/Rigid Body/Nonlinear Wave Elevation ==
  Displacement : Inport
  Time : Inport  Port=2
  Add : Sum  Inputs=+-
  Center of Gravity : Constant  Value=body.hydroData.properties.cg
  Constant : Constant  Value=[0 0 0]
  Linear or Instantaneous Free Surface : Subsystem  Variant=on
  Mux : Mux  Inputs=2
  Wave Elevation : Outport
  wires:
  Displacement/1 -> Add/1  "x"
  Linear or Instantaneous Free Surface/1(Out1) -> Wave Elevation/1
  Add/1 -> Linear or Instantaneous Free Surface/1(In1)  "x_cg"
  Mux/1 -> Add/2
  Center of Gravity/1 -> Mux/1  "cg"
  Constant/1 -> Mux/2
  Time/1 -> Linear or Instantaneous Free Surface/2(In2)
